simulink model "Tetris"  (R2023a)
settings: Solver=VariableStepAuto  StartTime=0.0  StopTime=inf  RelTol=1e-3  EnableMultiTasking=on
libraries: Miscellaneous x183, Byte_Multiplexers_Lib x77, Tetris_Lib x34, simulink_extras x11, Counters_Lib x7, Arithmetic_Operations_Lib x5, Word_Multiplexers_Lib x5, Decoders_Lib x4, Memory_Blocks_Lib x3, Bit_Multiplexers_Lib x2, dspobslib x1
(part 1 of 3)
settings Model: SnapshotBufferSize=2000  SnapshotInterval=1  PacingRate=79  Creator=Jozko Mrkvicka  LastModifiedBy=Jozko Mrkvicka
settings SolverCC: AlgebraicLoopSolver=TrustRegion
settings DataIOCC: ReturnWorkspaceOutputs=off
settings OptimizationCC: LifeSpan=inf
settings DebuggingCC: UnconnectedInputMsg=warning  UnconnectedOutputMsg=warning  UnconnectedLineMsg=warning  SFUnexpectedBacktrackingDiag=warning  SFNoUnconditionalDefaultTransitionDiag=warning  ArithmeticOperatorsInVariantConditions=warning
settings ModelReferenceCC: EnableRefExpFcnMdlSchedulingChecks=on
settings SFSimCC: SimUseLocalCustomCode=off  CustomCodeUndefinedFunction=UseInterfaceOnly
settings RTWCC: RTWUseLocalCustomCode=off
settings CodeAppCC: StateflowObjectComments=on
settings GRTTargetCC: TargetLangStandard=C89/C90 (ANSI)
settings ConfigComp: CovMetricSettings=dw  CovSaveCumulativeToWorkspaceVar=on  CovSaveSingleToWorkspaceVar=on  CovExternalEMLEnable=off

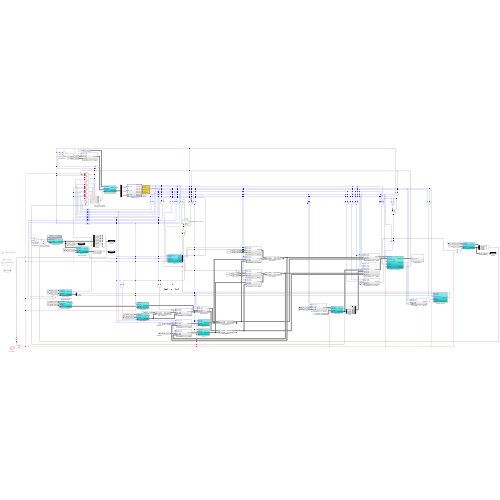
[thumbnail: Simulink's stored preview of the top-level diagram]
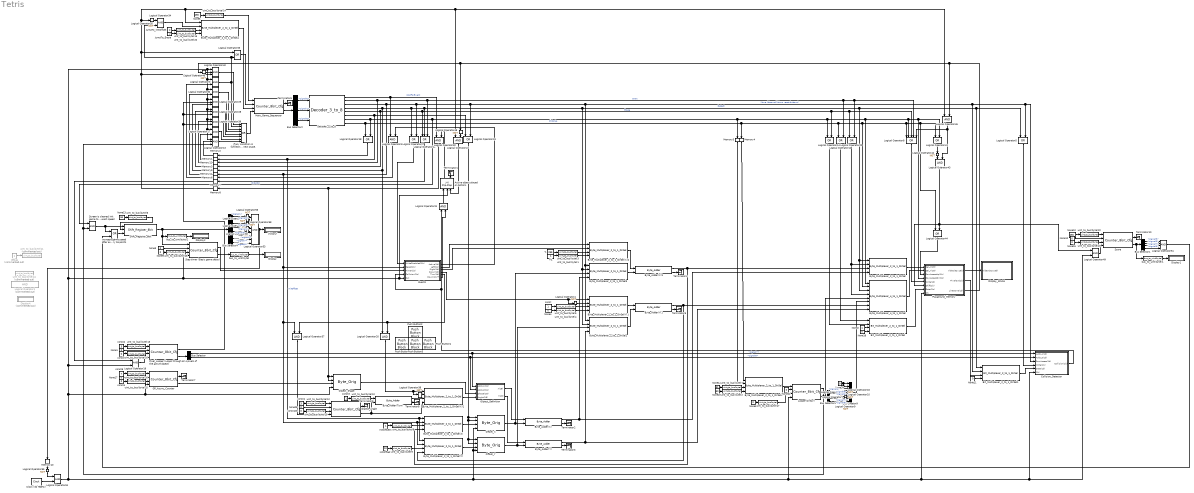
== system Tetris ==
  +1 : Constant  OutDataTypeStr=uint8
  -1 : Constant  Value=255  OutDataTypeStr=uint8
  "Active object placed on bottom " : simulink_extras/Flip Flops/J-K Flip-Flop  initial_condition=0
  Bit_Multiplexer_2_to_1_DirSel : Bit_Multiplexers_Lib/Bit_Multiplexers_Lib/Bit_Multiplexer_2_to_1_DirSel  SystemSampleTime=-1  VariantActivationTime=update diagram  Latency=0  AutoFrameSizeCalculation=off
  Bit_Multiplexer_2_to_1_DirSel1 : Bit_Multiplexers_Lib/Bit_Multiplexers_Lib/Bit_Multiplexer_2_to_1_DirSel  SystemSampleTime=-1  VariantActivationTime=update diagram  Latency=0  AutoFrameSizeCalculation=off
  Bus Creator9 : BusCreator  Inputs=8
  Bus Selector : BusSelector  OutputSignals=signal7,signal8
  Bus Selector1 : BusSelector  OutputSignals=signal5,signal6,signal7,signal8
  Bus Selector2 : BusSelector  OutputSignals=signal6,signal7,signal8
  Bus Selector3 : BusSelector  OutputSignals=signal4,signal5,signal6,signal7,signal8
  Bus Selector4 : BusSelector  OutputSignals=signal1,signal2,signal3,signal4,signal5,signal6,signal7,signal8
  Byte_Adder(Turn) : Arithmetic_Operations_Lib/Arithmetic_Operations_Lib/Byte_Adder  SystemSampleTime=-1  VariantActivationTime=update diagram  Latency=0  AutoFrameSizeCalculation=off
  Byte_Adder(X) : Arithmetic_Operations_Lib/Arithmetic_Operations_Lib/Byte_Adder  SystemSampleTime=-1  VariantActivationTime=update diagram  Latency=0  AutoFrameSizeCalculation=off
  Byte_Adder(X)1 : Arithmetic_Operations_Lib/Arithmetic_Operations_Lib/Byte_Adder  SystemSampleTime=-1  VariantActivationTime=update diagram  Latency=0  AutoFrameSizeCalculation=off
  Byte_Adder(Y) : Arithmetic_Operations_Lib/Arithmetic_Operations_Lib/Byte_Adder  SystemSampleTime=-1  VariantActivationTime=update diagram  Latency=0  AutoFrameSizeCalculation=off
  Byte_Adder(Y)1 : Arithmetic_Operations_Lib/Arithmetic_Operations_Lib/Byte_Adder  SystemSampleTime=-1  VariantActivationTime=update diagram  Latency=0  AutoFrameSizeCalculation=off
  Byte_Multiplexer_2_to_1_DirSel{,1..4} (5 alike) : Byte_Multiplexers_Lib/Byte_Multiplexers_Lib/Byte_Multiplexer_2_to_1_DirSel  SystemSampleTime=-1  VariantActivationTime=update diagram  Latency=0  AutoFrameSizeCalculation=off
  Byte_Multiplexer_2_to_1_DirSel(X) : Byte_Multiplexers_Lib/Byte_Multiplexers_Lib/Byte_Multiplexer_2_to_1_DirSel  SystemSampleTime=-1  VariantActivationTime=update diagram  Latency=0  AutoFrameSizeCalculation=off
  Byte_Multiplexer_2_to_1_DirSel(X)1 : Byte_Multiplexers_Lib/Byte_Multiplexers_Lib/Byte_Multiplexer_2_to_1_DirSel  SystemSampleTime=-1  VariantActivationTime=update diagram  Latency=0  AutoFrameSizeCalculation=off
  Byte_Multiplexer_2_to_1_DirSel(X)2 : Byte_Multiplexers_Lib/Byte_Multiplexers_Lib/Byte_Multiplexer_2_to_1_DirSel  SystemSampleTime=-1  VariantActivationTime=update diagram  Latency=0  AutoFrameSizeCalculation=off
  Byte_Multiplexer_2_to_1_DirSel(Y) : Byte_Multiplexers_Lib/Byte_Multiplexers_Lib/Byte_Multiplexer_2_to_1_DirSel  SystemSampleTime=-1  VariantActivationTime=update diagram  Latency=0  AutoFrameSizeCalculation=off
  Byte_Multiplexer_2_to_1_DirSel(Y)1 : Byte_Multiplexers_Lib/Byte_Multiplexers_Lib/Byte_Multiplexer_2_to_1_DirSel  SystemSampleTime=-1  VariantActivationTime=update diagram  Latency=0  AutoFrameSizeCalculation=off
  Byte_Multiplexer_4_to_1_DirSel : Byte_Multiplexers_Lib/Byte_Multiplexers_Lib/Byte_Multiplexer_4_to_1_DirSel  SystemSampleTime=-1  VariantActivationTime=update diagram  Latency=0  AutoFrameSizeCalculation=off
  Clock (32 768Hz) : simulink_extras/Flip Flops/Clock  period=1
  Collision_Detector : Subsystem
  Decoder_3_to_8 : Decoders_Lib/Decoders_Lib/Decoder_3_to_8  SystemSampleTime=-1  VariantActivationTime=update diagram  Latency=0  AutoFrameSizeCalculation=off
  Display : Display
  Display1 : Display
  Display2 : Display
  Display4 : Display  Commented=on
  Display_32x16 : Subsystem
  Events : Subsystem
  GP_Async_Counter : Counters_Lib/Counter_8bit_Cfg  SystemSampleTime=-1  VariantActivationTime=update diagram  Latency=0  AutoFrameSizeCalculation=off
  If any condition is fulfilled then we go to next state. : Logic  Operator=OR  Inputs=8  IconShape=distinctive  AllPortsSameDT=off  OutDataTypeStr=boolean
  Increase game speed after every 16 points : Logic  Operator=OR  IconShape=distinctive  OutDataTypeStr=boolean
  InitOffsetX : Constant  OutDataTypeStr=uint8
  InitOffsetY : Constant  Value=10  OutDataTypeStr=uint8
  "JumpTo_Erase     " : Constant  Value=3  OutDataTypeStr=uint8
  JumpTo_InitOffset : Constant  Value=2  OutDataTypeStr=uint8
  Logical Operator1 : Logic  Commented=on  Inputs=12  IconShape=distinctive  AllPortsSameDT=off  OutDataTypeStr=boolean
  Logical Operator{4,7,9..11,16,35,42,46,48,55..60} (16 alike) : Logic  Operator=NOT  Inputs=4  IconShape=distinctive  AllPortsSameDT=off  OutDataTypeStr=boolean
  Logical Operator{5,12,14,18,22..23,27,33,41,44} (10 alike) : Logic  Operator=OR  IconShape=distinctive  OutDataTypeStr=boolean
  Logical Operator{13,28..29,39..40} (5 alike) : Logic  Inputs=3  IconShape=distinctive  AllPortsSameDT=off  OutDataTypeStr=boolean
  Logical Operator{3,6,17,20,30..32,34,37,43,45,47,49,61} (14 alike) : Logic  IconShape=distinctive  AllPortsSameDT=off  OutDataTypeStr=boolean
  Logical Operator19 : Logic  IconShape=distinctive  AllPortsSameDT=off
  Logical Operator21 : Logic  Operator=OR  Inputs=3  IconShape=distinctive  AllPortsSameDT=off  OutDataTypeStr=boolean
  Logical Operator38 : Logic  Operator=NOT  IconShape=distinctive  AllPortsSameDT=off  OutDataTypeStr=boolean
  Logical Operator51 : Logic  Inputs=4  IconShape=distinctive  AllPortsSameDT=off  OutDataTypeStr=boolean
  Logical Operator53 : Logic  Inputs=8  IconShape=distinctive  AllPortsSameDT=off  OutDataTypeStr=boolean
  Logical Operator8 : Logic  Operator=OR  Inputs=5  IconShape=distinctive  OutDataTypeStr=boolean
  Looper(ClrScr) : Counters_Lib/Counter_8bit_Cfg  SystemSampleTime=-1  VariantActivationTime=update diagram  Latency=0  AutoFrameSizeCalculation=off
  Main_Game_Sequencer : Counters_Lib/Counter_8bit_Cfg  SystemSampleTime=-1  VariantActivationTime=update diagram  Latency=0  AutoFrameSizeCalculation=off
  Memory{1..12} (12 alike) : Memory
  None{1,3,11..12,17..18,22,24,28} (9 alike) : Constant  Value=0  OutDataTypeStr=boolean
  None10 : Constant  Value=255  OutDataTypeStr=uint8
  None13 : Constant  Value=64  OutDataTypeStr=uint8
  None14 : Constant  Value=31  OutDataTypeStr=uint8
  None{4,8..9,15} (4 alike) : Constant  Value=0  OutDataTypeStr=uint8
  None2 : Constant  OutDataTypeStr=boolean
  None23 : Constant  Value=30  OutDataTypeStr=uint8
  None5 : Constant  Value=255  OutDataTypeStr=uint8
  Object_Angle : Counters_Lib/Counter_8bit_Cfg  SystemSampleTime=-1  VariantActivationTime=update diagram  Latency=0  AutoFrameSizeCalculation=off
  Object_Definition : Subsystem
  Object_Shape : Memory_Blocks_Lib/Memory_Blocks_Lib/Byte_Orig  SystemSampleTime=-1  VariantActivationTime=update diagram  Latency=0  AutoFrameSizeCalculation=off
  Offset_X : Memory_Blocks_Lib/Memory_Blocks_Lib/Byte_Orig  SystemSampleTime=-1  VariantActivationTime=update diagram  Latency=0  AutoFrameSizeCalculation=off
  Offset_Y : Memory_Blocks_Lib/Memory_Blocks_Lib/Byte_Orig  SystemSampleTime=-1  VariantActivationTime=update diagram  Latency=0  AutoFrameSizeCalculation=off
  Pixel_Looper (Loops through all 4 pixels of the active object) : Counters_Lib/Counter_8bit_Cfg  SystemSampleTime=-1  VariantActivationTime=update diagram  Latency=0  AutoFrameSizeCalculation=off
  Playground_Memory : Subsystem
  Push Button : PushButtonBlock  ButtonText=Left  OffValue=0.000000
  Push Button1 : PushButtonBlock  ButtonText=Right  OffValue=0.000000
  Push Button2 : PushButtonBlock  ButtonText=Turn  OffValue=0.000000
  Push Button3 : PushButtonBlock  ButtonText=Down  OffValue=0.000000
  Score : Counters_Lib/Counter_8bit_Cfg  SystemSampleTime=-1  VariantActivationTime=update diagram  Latency=0  AutoFrameSizeCalculation=off
  Screen is cleared; Init game to slowest speed : Logic  IconShape=distinctive  AllPortsSameDT=off  OutDataTypeStr=boolean
  Shift_Register_8bit : Tetris_Lib/Shift_Register_8bit  SystemSampleTime=-1  VariantActivationTime=update diagram  Latency=0  AutoFrameSizeCalculation=off
  Step timer (Basic game delay) : Counters_Lib/Counter_8bit_Cfg  SystemSampleTime=-1  VariantActivationTime=update diagram  Latency=0  AutoFrameSizeCalculation=off
  Terminator{1..10} (10 alike) : Terminator
  Victory! : Display
  bus_to_uint(byte) : Miscellaneous/bus_to_uint(byte)  SystemSampleTime=-1  VariantActivationTime=update diagram  Latency=0  AutoFrameSizeCalculation=off
  bus_to_uint(byte)1 : Miscellaneous/bus_to_uint(byte)  SystemSampleTime=-1  VariantActivationTime=update diagram  Latency=0  AutoFrameSizeCalculation=off
  bus_to_uint(byte)2 : Miscellaneous/bus_to_uint(byte)  SystemSampleTime=-1  VariantActivationTime=update diagram  Latency=0  AutoFrameSizeCalculation=off
  const : Constant  OutDataTypeStr=uint8
  const1 : Constant  Value=3  OutDataTypeStr=uint8
  const100 : Constant  Value=0  OutDataTypeStr=uint8
  const2 : Constant  Value=3  OutDataTypeStr=uint8
  const3 : Constant  OutDataTypeStr=uint8
  const4 : Constant  Value=0  OutDataTypeStr=uint8
  const5 : Constant  Value=0  OutDataTypeStr=uint8
  const6 : Constant  Value=7  OutDataTypeStr=uint8
  debug : Constant  Commented=on  OutDataTypeStr=uint8
  uint_to_bus(byte){1..10,12..20,22..23,25..26} (23 alike) : Miscellaneous/uint_to_bus(byte)  SystemSampleTime=-1  VariantActivationTime=update diagram  Latency=0  AutoFrameSizeCalculation=off
  uint_to_bus(byte)11 : Miscellaneous/uint_to_bus(byte)  Commented=on  SystemSampleTime=-1  VariantActivationTime=update diagram  Latency=0  AutoFrameSizeCalculation=off
  uint_to_bus(byte)24 : Miscellaneous/uint_to_bus(byte)  Commented=on  SystemSampleTime=-1  VariantActivationTime=update diagram  Latency=0  AutoFrameSizeCalculation=off
  wires:
  None1/1 -> Pixel_Looper (Loops through all 4 pixels of the active object)/2
  Playground_Memory/2(PixelOut(1b)) -> Bit_Multiplexer_2_to_1_DirSel1/3
  Playground_Memory/1(Video(32x16b)) -> Display_32x16/1(Video(32x16b))
  Offset_Y/1 -> Byte_Multiplexer_2_to_1_DirSel2/3, Byte_Adder(Y)/2
  Offset_X/1 -> Byte_Multiplexer_2_to_1_DirSel3/3, Byte_Adder(X)/2
  Bit_Multiplexer_2_to_1_DirSel/1 -> Playground_Memory/7(Data(1b))
  Pixel_Looper (Loops through all 4 pixels of the active object)/2 -> Bus Selector/1
  uint_to_bus(byte)13/1 -> Pixel_Looper (Loops through all 4 pixels of the active object)/1
  Byte_Adder(X)/2 -> Terminator2/1
  Byte_Adder(Y)/2 -> Terminator3/1
  uint_to_bus(byte)4/1 -> Byte_Multiplexer_2_to_1_DirSel(Y)1/4
  uint_to_bus(byte)5/1 -> Byte_Multiplexer_2_to_1_DirSel(Y)1/3
  Bus Selector/1 -> Collision_Detector/1(Addr_1(1b)), Object_Definition/1(Addr_1(1b))  "<signal7>"
  Bus Selector/2 -> Collision_Detector/2(Addr_0(1b)), Object_Definition/2(Addr_0(1b))  "<signal8>"
  Decoder_3_to_8/4 -> Logical Operator5/1, Bit_Multiplexer_2_to_1_DirSel1/1, Byte_Multiplexer_4_to_1_DirSel/3, Byte_Multiplexer_2_to_1_DirSel/1, Byte_Multiplexer_2_to_1_DirSel3/2, Byte_Multiplexer_2_to_1_DirSel2/2, Logical Operator21/2, Logical Operator27/1, Memory9/1, Logical Operator20/1  "Detect"
  Decoder_3_to_8/3 -> Collision_Detector/3(RowAccess(1b)), Logical Operator5/2, Bit_Multiplexer_2_to_1_DirSel1/2, Byte_Multiplexer_2_to_1_DirSel2/1, Byte_Multiplexer_2_to_1_DirSel3/1, Logical Operator23/2, Logical Operator27/2, Logical Operator37/1, Byte_Multiplexer_2_to_1_DirSel(X)/2, Byte_Multiplexer_2_to_1_DirSel(Y)/2, Events/2(Reset(1b)), Memory11/1  "Move (clear collisions, reset buttons)"
  None2/1 -> Bit_Multiplexer_2_to_1_DirSel/3
  None18/1 -> Bit_Multiplexer_2_to_1_DirSel/4
  Logical Operator8/1 -> Playground_Memory/5(Write(1b))
  Decoder_3_to_8/5 -> Logical Operator8/3, Logical Operator22/1, Logical Operator14/2, Logical Operator21/1, Memory3/1  "Erase"
  Byte_Multiplexer_2_to_1_DirSel(X)2/1 -> Byte_Adder(X)1/1
  Byte_Multiplexer_2_to_1_DirSel(Y)1/1 -> Byte_Adder(Y)1/1
  Byte_Multiplexer_2_to_1_DirSel/1 -> Playground_Memory/1(Sel_X(1B))
  Byte_Multiplexer_4_to_1_DirSel/1 -> Playground_Memory/2(Sel_Y(1B))
  Byte_Adder(X)/1 -> Byte_Multiplexer_2_to_1_DirSel3/4, Byte_Multiplexer_2_to_1_DirSel/4
  Byte_Adder(Y)/1 -> Byte_Multiplexer_2_to_1_DirSel2/4, Byte_Multiplexer_4_to_1_DirSel/8
  Object_Definition/1(X(1B)) -> Byte_Adder(X)/1
  Object_Definition/2(Y(1B)) -> Byte_Adder(Y)/1
  Byte_Multiplexer_2_to_1_DirSel(Y)/1 -> Offset_Y/3
  Byte_Multiplexer_2_to_1_DirSel(X)/1 -> Offset_X/3
  None11/1 -> Bit_Multiplexer_2_to_1_DirSel1/4
  Logical Operator5/1 -> Collision_Detector/4(Write(1b))
  Bus Selector2/2 -> Decoder_3_to_8/2  "<signal7>"
  Main_Game_Sequencer/2 -> Bus Selector2/1
  Bus Selector2/3 -> Decoder_3_to_8/3  "<signal8>"
  Decoder_3_to_8/6 -> Logical Operator23/1, Memory1/1, Byte_Multiplexer_2_to_1_DirSel(X)/1, Byte_Multiplexer_2_to_1_DirSel(Y)/1  "InitOffset"
  Decoder_3_to_8/8 -> Memory4/1, Byte_Multiplexer_4_to_1_DirSel/2, Logical Operator44/1, Logical Operator41/1, Logical Operator8/1, Logical Operator12/1, Logical Operator18/1  "ClrScrUp"
  If any condition is fulfilled then we go to next state./1 -> Main_Game_Sequencer/4
  None23/1 -> uint_to_bus(byte)2/1
  None22/1 -> Looper(ClrScr)/2
  None24/1 -> Bus Creator9/3, Bus Creator9/2, Bus Creator9/1
  Bus Creator9/1 -> Byte_Multiplexer_4_to_1_DirSel/6
  Decoder_3_to_8/7 -> Screen is cleared; Init game to slowest speed/1, Byte_Multiplexer_4_to_1_DirSel/1, Logical Operator41/2, Playground_Memory/4(RowAccessDn(1b)), Logical Operator8/2, Logical Operator14/1, Memory5/1, Logical Operator18/2  "ClrScrDn"
  Logical Operator9/1 -> Bus Creator9/8
  Logical Operator7/1 -> Bus Creator9/7
  Logical Operator10/1 -> Bus Creator9/6
  Logical Operator11/1 -> Bus Creator9/5
  Logical Operator13/1 -> If any condition is fulfilled then we go to next state./8
  Looper(ClrScr)/1 -> Logical Operator13/3, Screen is cleared; Init game to slowest speed/2
  Collision_Detector/1(Collision(1b)) -> Events/4(Collision(1b)), Logical Operator31/1
  Logical Operator12/1 -> Bit_Multiplexer_2_to_1_DirSel/1
  Looper(ClrScr)/2 -> Byte_Multiplexer_4_to_1_DirSel/5, Bus Selector3/1
  Logical Operator14/1 -> Bit_Multiplexer_2_to_1_DirSel/2
  Logical Operator16/1 -> Bus Creator9/4
  Bus Selector3/1 -> Logical Operator16/1  "<signal4>"
  Bus Selector3/2 -> Logical Operator11/1  "<signal5>"
  Bus Selector3/3 -> Logical Operator10/1  "<signal6>"
  Bus Selector3/4 -> Logical Operator7/1  "<signal7>"
  Bus Selector3/5 -> Logical Operator9/1  "<signal8>"
  Logical Operator17/1 -> If any condition is fulfilled then we go to next state./7
  Logical Operator18/1 -> Memory2/1
  Logical Operator19/1 -> Pixel_Looper (Loops through all 4 pixels of the active object)/4
  Logical Operator22/1 -> Byte_Multiplexer_4_to_1_DirSel/4, Byte_Multiplexer_2_to_1_DirSel/2
  Logical Operator4/1 -> Byte_Multiplexer_2_to_1_DirSel(Y)1/2
  +1/1 -> uint_to_bus(byte)1/1
  uint_to_bus(byte)1/1 -> Byte_Multiplexer_2_to_1_DirSel(X)2/4
  -1/1 -> uint_to_bus(byte)3/1
  uint_to_bus(byte)3/1 -> Byte_Multiplexer_2_to_1_DirSel(X)2/3
  None4/1 -> uint_to_bus(byte)4/1
  const/1 -> uint_to_bus(byte)5/1
  uint_to_bus(byte)6/1 -> Shift_Register_8bit/2
  None13/1 -> uint_to_bus(byte)6/1
  None3/1 -> Step timer (Basic game delay)/2
  Byte_Multiplexer_2_to_1_DirSel1/1 -> Looper(ClrScr)/1
  uint_to_bus(byte)2/1 -> Byte_Multiplexer_2_to_1_DirSel1/4
  None14/1 -> uint_to_bus(byte)7/1
  uint_to_bus(byte)7/1 -> Byte_Multiplexer_2_to_1_DirSel1/3
  Memory4/1 -> Byte_Multiplexer_2_to_1_DirSel1/1
  Memory5/1 -> Byte_Multiplexer_2_to_1_DirSel1/2
  None28/1 -> Object_Angle/2
  InitOffsetX/1 -> uint_to_bus(byte)8/1
  InitOffsetY/1 -> uint_to_bus(byte)9/1
  uint_to_bus(byte)8/1 -> Byte_Multiplexer_2_to_1_DirSel(X)/3
  uint_to_bus(byte)9/1 -> Byte_Multiplexer_2_to_1_DirSel(Y)/3
  Pixel_Looper (Loops through all 4 pixels of the active object)/1 -> Logical Operator39/3, Logical Operator28/3, Logical Operator29/2
  Memory7/1 -> Logical Operator19/1
  Logical Operator21/1 -> Memory7/1
  Events/2(Left(1b)) -> Byte_Multiplexer_2_to_1_DirSel(X)2/1
  Events/3(Right(1b)) -> Byte_Multiplexer_2_to_1_DirSel(X)2/2
  Bit_Multiplexer_2_to_1_DirSel1/1 -> Collision_Detector/5(Data(1b))
  Logical Operator23/1 -> Offset_Y/2, Offset_Y/1, Offset_X/2, Offset_X/1
  Logical Operator27/1 -> Events/1(WriteDisabled(1b))
  Byte_Adder(Y)1/1 -> Byte_Multiplexer_4_to_1_DirSel/7, Byte_Multiplexer_2_to_1_DirSel(Y)/4
  Byte_Adder(X)1/1 -> Byte_Multiplexer_2_to_1_DirSel/3, Byte_Multiplexer_2_to_1_DirSel(X)/4
  Byte_Adder(X)1/2 -> Terminator4/1
  Byte_Adder(Y)1/2 -> Terminator5/1
  Byte_Multiplexer_2_to_1_DirSel3/1 -> Byte_Adder(X)1/2
  Byte_Multiplexer_2_to_1_DirSel2/1 -> Byte_Adder(Y)1/2
  Decoder_3_to_8/2 -> Memory12/1, Logical Operator12/2, Logical Operator22/2, Logical Operator8/4, Logical Operator21/3  "Draw"
  Bus Selector2/1 -> Decoder_3_to_8/1  "<signal6>"
  Events/4(Down(1b)) -> Byte_Multiplexer_2_to_1_DirSel(Y)1/1, Logical Operator4/1
  Events/5(Turn(1b)) -> Logical Operator37/2, Logical Operator20/2
  const3/1 -> uint_to_bus(byte)10/1
  uint_to_bus(byte)10/1 -> Byte_Adder(Turn)/1
  Object_Angle/2 -> Byte_Adder(Turn)/2, Byte_Multiplexer_2_to_1_DirSel(X)1/4
  Byte_Adder(Turn)/2 -> Terminator8/1
  Byte_Adder(Turn)/1 -> Byte_Multiplexer_2_to_1_DirSel(X)1/3
  Byte_Multiplexer_2_to_1_DirSel(X)1/1 -> Object_Definition/4(Angle(1B))
  Logical Operator37/1 -> Object_Angle/4
  Logical Operator20/1 -> Logical Operator38/1, Byte_Multiplexer_2_to_1_DirSel(X)1/1
  Logical Operator38/1 -> Byte_Multiplexer_2_to_1_DirSel(X)1/2
  Logical Operator61/1 -> Logical Operator19/2, Logical Operator40/1, Logical Operator13/1, Logical Operator17/1, Logical Operator39/1, Logical Operator28/1, Logical Operator29/1, Logical Operator30/1, Logical Operator3/1, Step timer (Basic game delay)/4, "Active object placed on bottom "/2, Events/5(CLK), Object_Shape/4, GP_Async_Counter/4, Looper(ClrScr)/4, Collision_Detector/6(CLK), Logical Operator49/2, Playground_Memory/8(Clk), Offset_X/4, Offset_Y/4
  const1/1 -> uint_to_bus(byte)12/1
  uint_to_bus(byte)12/1 -> Object_Angle/1
  Object_Angle/1 -> Terminator9/1
  const2/1 -> uint_to_bus(byte)13/1
  None5/1 -> uint_to_bus(byte)14/1
  uint_to_bus(byte)14/1 -> Main_Game_Sequencer/1
  Byte_Multiplexer_2_to_1_DirSel4/1 -> Main_Game_Sequencer/3
  "JumpTo_Erase     "/1 -> uint_to_bus(byte)20/1
  const5/1 -> uint_to_bus(byte)16/1
  uint_to_bus(byte)16/1 -> Pixel_Looper (Loops through all 4 pixels of the active object)/3
  None8/1 -> uint_to_bus(byte)17/1
  uint_to_bus(byte)17/1 -> Looper(ClrScr)/3
  uint_to_bus(byte)18/1 -> Step timer (Basic game delay)/3
  None9/1 -> uint_to_bus(byte)18/1
  const100/1 -> uint_to_bus(byte)19/1
  uint_to_bus(byte)19/1 -> Object_Angle/3
  Logical Operator28/1 -> If any condition is fulfilled then we go to next state./5
  Logical Operator29/1 -> If any condition is fulfilled then we go to next state./4
  Logical Operator30/1 -> If any condition is fulfilled then we go to next state./3
  Memory2/1 -> Logical Operator13/2
  Memory12/1 -> Logical Operator39/2
  Memory3/1 -> Logical Operator28/2
  Memory9/1 -> Logical Operator29/3
  Memory1/1 -> Logical Operator17/2
  Decoder_3_to_8/1 -> Logical Operator32/1, Logical Operator6/1  "WaitForEvent"
  Main_Game_Sequencer/1 -> Terminator6/1
  Memory11/1 -> Logical Operator30/2
  Step timer (Basic game delay)/2 -> bus_to_uint(byte)/1
  Logical Operator6/1 -> Memory6/1
  Logical Operator3/1 -> Logical Operator33/2, Logical Operator34/2, If any condition is fulfilled then we go to next state./2
  Logical Operator39/1 -> If any condition is fulfilled then we go to next state./6
  Step timer (Basic game delay)/1 -> Events/3(Timer(1b))
  bus_to_uint(byte)/1 -> Display/1
  Events/1(Active(1b)) -> Logical Operator6/2
  Memory6/1 -> Logical Operator3/2
  Logical Operator31/1 -> "Active object placed on bottom "/1
  "Active object placed on bottom "/1 -> Logical Operator32/2
  JumpTo_InitOffset/1 -> uint_to_bus(byte)15/1
  uint_to_bus(byte)15/1 -> Byte_Multiplexer_2_to_1_DirSel4/3
  uint_to_bus(byte)20/1 -> Byte_Multiplexer_2_to_1_DirSel4/4
  Logical Operator33/1 -> Main_Game_Sequencer/2
  Logical Operator34/1 -> Byte_Multiplexer_2_to_1_DirSel4/2
  Logical Operator35/1 -> Logical Operator34/1
  Logical Operator40/1 -> If any condition is fulfilled then we go to next state./1
  Playground_Memory/3(LineDone(1b)) -> Logical Operator46/1, Logical Operator48/1, Logical Operator45/2
  Logical Operator41/1 -> Logical Operator42/1
  Logical Operator42/1 -> Logical Operator43/1
  Logical Operator44/1 -> Playground_Memory/3(RowAccessUp(1b))
  Logical Operator45/1 -> Logical Operator8/5, Logical Operator43/2
  Logical Operator46/1 -> Logical Operator40/2
  Logical Operator47/1 -> "Active object placed on bottom "/3
  Logical Operator48/1 -> Logical Operator47/2
  None10/1 -> uint_to_bus(byte)22/1
  uint_to_bus(byte)22/1 -> Score/1
  None12/1 -> Score/2
  bus_to_uint(byte)1/1 -> Display1/1
  Score/2 -> bus_to_uint(byte)1/1, Bus Selector1/1
  Logical Operator43/1 -> Playground_Memory/6(Shift(1b)), Logical Operator49/1, Logical Operator44/2
  uint_to_bus(byte)23/1 -> Score/3
  None15/1 -> uint_to_bus(byte)23/1
  Logical Operator49/1 -> Score/4
  Shift_Register_8bit/1 -> Step timer (Basic game delay)/1, bus_to_uint(byte)2/1, Bus Selector4/1
  Screen is cleared; Init game to slowest speed/1 -> Shift_Register_8bit/1, Increase game speed after every 16 points/1
  Bus Selector1/1 -> Logical Operator51/1  "<signal5>"
  Bus Selector1/3 -> Logical Operator51/3  "<signal7>"
  Bus Selector1/2 -> Logical Operator51/2  "<signal6>"
  Bus Selector1/4 -> Logical Operator51/4  "<signal8>"
  Logical Operator51/1 -> Increase game speed after every 16 points/2
  Increase game speed after every 16 points/1 -> Shift_Register_8bit/3
  bus_to_uint(byte)2/1 -> Display2/1
  Bus Selector4/1 -> Logical Operator56/1  "<signal1>"
  Bus Selector4/2 -> Logical Operator57/1  "<signal2>"
  Bus Selector4/3 -> Logical Operator58/1  "<signal3>"
  Bus Selector4/4 -> Logical Operator59/1  "<signal4>"
  Logical Operator56/1 -> Logical Operator53/1
  Logical Operator57/1 -> Logical Operator53/2
  Logical Operator58/1 -> Logical Operator53/3
  Logical Operator59/1 -> Logical Operator53/4
  Bus Selector4/5 -> Logical Operator60/1  "<signal5>"
  Bus Selector4/6 -> Logical Operator53/6  "<signal6>"
  Bus Selector4/7 -> Logical Operator53/7  "<signal7>"
  Bus Selector4/8 -> Logical Operator53/8  "<signal8>"
  Logical Operator60/1 -> Logical Operator53/5
  Logical Operator53/1 -> Victory!/1, Memory10/1
  Clock (32 768Hz)/1 -> Logical Operator61/2
  Logical Operator55/1 -> Logical Operator61/1
  Memory10/1 -> Logical Operator55/1
  Memory8/1 -> Logical Operator45/1, Logical Operator47/1, Byte_Multiplexer_2_to_1_DirSel4/1, Logical Operator35/1, Logical Operator33/1, Logical Operator40/3
  "Active object placed on bottom "/2 -> Terminator1/1
  Object_Shape/1 -> Object_Definition/3(Shape(1B))
  debug/1 -> uint_to_bus(byte)11/1
  const4/1 -> uint_to_bus(byte)25/1
  None17/1 -> GP_Async_Counter/2
  uint_to_bus(byte)25/1 -> GP_Async_Counter/3
  uint_to_bus(byte)26/1 -> GP_Async_Counter/1
  const6/1 -> uint_to_bus(byte)26/1
  GP_Async_Counter/2 -> Object_Shape/3
  GP_Async_Counter/1 -> Terminator7/1
  Score/1 -> Terminator10/1
  Logical Operator32/1 -> Memory8/1, Object_Shape/1, Object_Shape/2
  Events/6(Down(1b)+) -> Logical Operator31/2

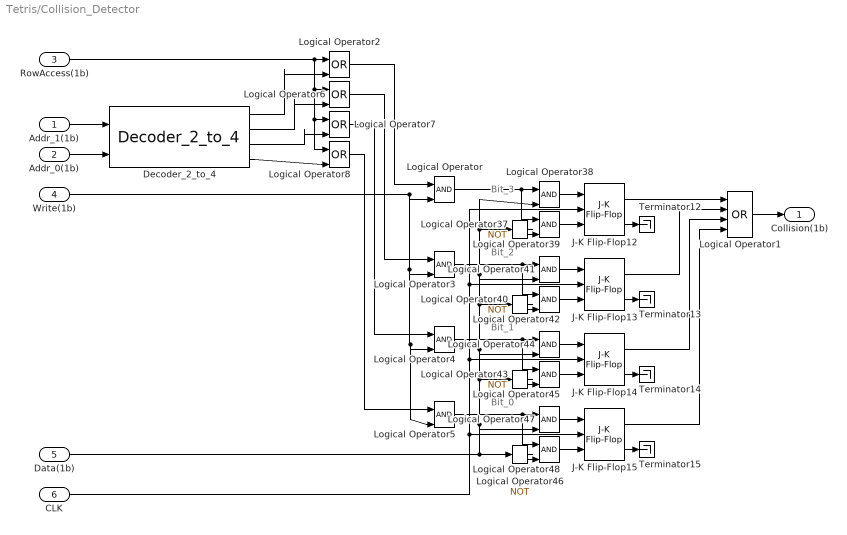
== system Tetris/Collision_Detector ==
  note: Bit_0
  note: Bit_1
  note: Bit_2
  note: Bit_3
  Addr_1(1b) : Inport
  Addr_0(1b) : Inport  Port=2
  RowAccess(1b) : Inport  Port=3
  Write(1b) : Inport  Port=4
  Data(1b) : Inport  Port=5
  CLK : Inport  Port=6
  Decoder_2_to_4 : Decoders_Lib/Decoders_Lib/Decoder_2_to_4  SystemSampleTime=-1  VariantActivationTime=update diagram  Latency=0  AutoFrameSizeCalculation=off
  J-K Flip-Flop{12..15} (4 alike) : simulink_extras/Flip Flops/J-K Flip-Flop  initial_condition=0
  Logical Operator{,3..5,38..39,41..42,44..45,47..48} (12 alike) : Logic  IconShape=distinctive  AllPortsSameDT=off  OutDataTypeStr=boolean
  Logical Operator1 : Logic  Operator=OR  Inputs=4  IconShape=distinctive  AllPortsSameDT=off  OutDataTypeStr=boolean
  Logical Operator{2,6..8} (4 alike) : Logic  Operator=OR  IconShape=distinctive  AllPortsSameDT=off  OutDataTypeStr=boolean
  Logical Operator{37,40,43,46} (4 alike) : Logic  Operator=NOT  IconShape=distinctive  AllPortsSameDT=off  OutDataTypeStr=boolean
  Terminator{12..15} (4 alike) : Terminator
  Collision(1b) : Outport
  wires:
  Logical Operator38/1 -> J-K Flip-Flop12/1
  J-K Flip-Flop12/2 -> Terminator12/1
  CLK/1 -> J-K Flip-Flop15/2, J-K Flip-Flop14/2, J-K Flip-Flop12/2, J-K Flip-Flop13/2
  Logical Operator37/1 -> Logical Operator39/2
  Logical Operator43/1 -> Logical Operator45/2
  J-K Flip-Flop14/1 -> Logical Operator1/3
  Logical Operator39/1 -> J-K Flip-Flop12/3
  J-K Flip-Flop12/1 -> Logical Operator1/1
  J-K Flip-Flop13/1 -> Logical Operator1/2
  Logical Operator42/1 -> J-K Flip-Flop13/3
  Logical Operator40/1 -> Logical Operator42/2
  Logical Operator47/1 -> J-K Flip-Flop15/1
  Logical Operator45/1 -> J-K Flip-Flop14/3
  Logical Operator44/1 -> J-K Flip-Flop14/1
  Data(1b)/1 -> Logical Operator38/2, Logical Operator37/1, Logical Operator41/2, Logical Operator40/1, Logical Operator44/2, Logical Operator43/1, Logical Operator47/2, Logical Operator46/1
  Logical Operator48/1 -> J-K Flip-Flop15/3
  J-K Flip-Flop15/2 -> Terminator15/1
  J-K Flip-Flop15/1 -> Logical Operator1/4
  J-K Flip-Flop14/2 -> Terminator14/1
  Write(1b)/1 -> Logical Operator/2, Logical Operator3/2, Logical Operator4/2, Logical Operator5/2
  J-K Flip-Flop13/2 -> Terminator13/1
  Logical Operator41/1 -> J-K Flip-Flop13/1
  Logical Operator46/1 -> Logical Operator48/2
  Logical Operator1/1 -> Collision(1b)/1
  Addr_0(1b)/1 -> Decoder_2_to_4/2
  Addr_1(1b)/1 -> Decoder_2_to_4/1
  Logical Operator5/1 -> Logical Operator47/1, Logical Operator48/1
  Logical Operator4/1 -> Logical Operator44/1, Logical Operator45/1
  Logical Operator3/1 -> Logical Operator41/1, Logical Operator42/1
  Logical Operator/1 -> Logical Operator39/1, Logical Operator38/1
  Logical Operator2/1 -> Logical Operator/1
  Logical Operator6/1 -> Logical Operator3/1
  Logical Operator7/1 -> Logical Operator4/1
  Logical Operator8/1 -> Logical Operator5/1
  Decoder_2_to_4/1 -> Logical Operator2/2
  Decoder_2_to_4/2 -> Logical Operator6/2
  Decoder_2_to_4/3 -> Logical Operator7/2
  Decoder_2_to_4/4 -> Logical Operator8/2
  RowAccess(1b)/1 -> Logical Operator2/1, Logical Operator6/1, Logical Operator7/1, Logical Operator8/1

== system Tetris/Display_32x16 ==
  note: Individual words in video memory are interpreted as columns by the Matrix Concatenate block in the following way:
      | - Word with the highest address is interpreted as the left-most column.
      | - Word with the lowest address is interpreted as the right-most column.
      | - MSB bit is interpreted as the top pixel of a particular column.
      | - LSB bit is interpreted as the bottom pixel of a particular column.
      |
      | On screen we want to interpret the words as rows (to correspond to the memory layout) in the following way:
      | - Word with highest address represents top row.
      | - Word with lowest address represents bottom row.
      | - MSB bit represents left-most pixel.
      | - LSB bit represents right-most pixel.
      |
      | To achieve this the Permute Dimensions block is utilized.
  Video(32x16b) : Inport
  Bus Selector1 : BusSelector  OutputSignals=signal1,signal2,signal3,signal4,signal5,signal6,signal7,signal8,signal9,signal10,signal11,signal12,signal13,signal14,signal15,signal16,signal17,signal18,signal19,signal20,signal21,signal22,signal23,signal24,signal25,signal26,signal27,signal28,signal29,signal30,signal31,signal32
  Matrix Concatenate6 : Concatenate  NumInputs=32  Mode=Multidimensional array  ConcatenateDimension=2
  Matrix Viewer2 : dspobslib/Matrix Viewer  ImageParams=off  CMapStr=[0 0.3 0; 0 1 0]  AxisColorbar=on  AxisParams=off  AxisOrigin=Upper left corner  AxisTickMode=Auto  XTickRange=[0 1]  YTickRange=[0 1]  XLabel=X-axis  YLabel=Y-axis  ZLabel=Z-axis  FigPos=[1700 10 200 400]  AxisZoom=on
      settings: YMin=0  YMax=1
  Permute Dimensions : PermuteDimensions
  wires:
  Matrix Concatenate6/1 -> Permute Dimensions/1
  Video(32x16b)/1 -> Bus Selector1/1
  Bus Selector1/9 -> Matrix Concatenate6/9  "<signal9>"
  Bus Selector1/1 -> Matrix Concatenate6/1  "<signal1>"
  Bus Selector1/2 -> Matrix Concatenate6/2  "<signal2>"
  Bus Selector1/32 -> Matrix Concatenate6/32  "<signal32>"
  Bus Selector1/31 -> Matrix Concatenate6/31  "<signal31>"
  Bus Selector1/30 -> Matrix Concatenate6/30  "<signal30>"
  Bus Selector1/29 -> Matrix Concatenate6/29  "<signal29>"
  Bus Selector1/28 -> Matrix Concatenate6/28  "<signal28>"
  Bus Selector1/27 -> Matrix Concatenate6/27  "<signal27>"
  Bus Selector1/26 -> Matrix Concatenate6/26  "<signal26>"
  Bus Selector1/25 -> Matrix Concatenate6/25  "<signal25>"
  Bus Selector1/3 -> Matrix Concatenate6/3  "<signal3>"
  Bus Selector1/4 -> Matrix Concatenate6/4  "<signal4>"
  Bus Selector1/5 -> Matrix Concatenate6/5  "<signal5>"
  Bus Selector1/6 -> Matrix Concatenate6/6  "<signal6>"
  Bus Selector1/7 -> Matrix Concatenate6/7  "<signal7>"
  Bus Selector1/8 -> Matrix Concatenate6/8  "<signal8>"
  Bus Selector1/10 -> Matrix Concatenate6/10  "<signal10>"
  Bus Selector1/11 -> Matrix Concatenate6/11  "<signal11>"
  Bus Selector1/12 -> Matrix Concatenate6/12  "<signal12>"
  Bus Selector1/13 -> Matrix Concatenate6/13  "<signal13>"
  Bus Selector1/14 -> Matrix Concatenate6/14  "<signal14>"
  Bus Selector1/15 -> Matrix Concatenate6/15  "<signal15>"
  Bus Selector1/16 -> Matrix Concatenate6/16  "<signal16>"
  Bus Selector1/17 -> Matrix Concatenate6/17  "<signal17>"
  Bus Selector1/18 -> Matrix Concatenate6/18  "<signal18>"
  Bus Selector1/19 -> Matrix Concatenate6/19  "<signal19>"
  Bus Selector1/20 -> Matrix Concatenate6/20  "<signal20>"
  Bus Selector1/21 -> Matrix Concatenate6/21  "<signal21>"
  Bus Selector1/22 -> Matrix Concatenate6/22  "<signal22>"
  Bus Selector1/23 -> Matrix Concatenate6/23  "<signal23>"
  Bus Selector1/24 -> Matrix Concatenate6/24  "<signal24>"
  Permute Dimensions/1 -> Matrix Viewer2/1

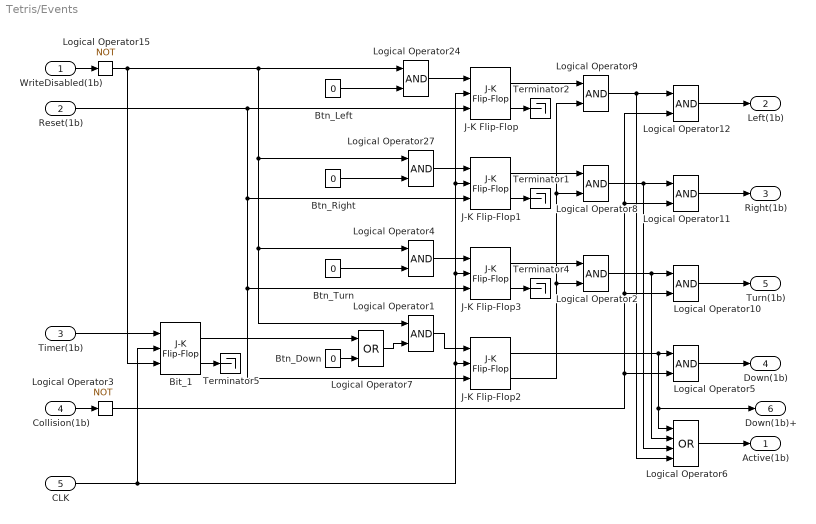
== system Tetris/Events ==
  WriteDisabled(1b) : Inport
  Reset(1b) : Inport  Port=2
  Timer(1b) : Inport  Port=3
  Collision(1b) : Inport  Port=4
  CLK : Inport  Port=5
  Bit_1 : simulink_extras/Flip Flops/J-K Flip-Flop  initial_condition=0
  Btn_Down : Constant  Value=0  OutDataTypeStr=boolean
  Btn_Left : Constant  Value=0  OutDataTypeStr=boolean
  Btn_Right : Constant  Value=0  OutDataTypeStr=boolean
  Btn_Turn : Constant  Value=0  OutDataTypeStr=boolean
  J-K Flip-Flop{,1..3} (4 alike) : simulink_extras/Flip Flops/J-K Flip-Flop  initial_condition=0
  Logical Operator{1..2,4..5,8..12,24,27} (11 alike) : Logic  IconShape=distinctive  AllPortsSameDT=off  OutDataTypeStr=boolean
  Logical Operator15 : Logic  Operator=NOT  Inputs=4  IconShape=distinctive  AllPortsSameDT=off  OutDataTypeStr=boolean
  Logical Operator3 : Logic  Operator=NOT  Inputs=4  IconShape=distinctive  AllPortsSameDT=off  OutDataTypeStr=boolean
  Logical Operator6 : Logic  Operator=OR  Inputs=4  IconShape=distinctive  AllPortsSameDT=off  OutDataTypeStr=boolean
  Logical Operator7 : Logic  Operator=OR  IconShape=distinctive  AllPortsSameDT=off  OutDataTypeStr=boolean
  Terminator{1..2,4..5} (4 alike) : Terminator
  Active(1b) : Outport
  Left(1b) : Outport  Port=2
  Right(1b) : Outport  Port=3
  Down(1b) : Outport  Port=4
  Turn(1b) : Outport  Port=5
  Down(1b)+ : Outport  Port=6
  wires:
  J-K Flip-Flop1/1 -> Logical Operator8/1
  J-K Flip-Flop/2 -> Terminator2/1
  Logical Operator27/1 -> J-K Flip-Flop1/1
  Btn_Right/1 -> Logical Operator27/2
  J-K Flip-Flop1/2 -> Terminator1/1
  CLK/1 -> J-K Flip-Flop3/2, J-K Flip-Flop1/2, J-K Flip-Flop/2, J-K Flip-Flop2/2, Bit_1/2
  Btn_Left/1 -> Logical Operator24/2
  Logical Operator24/1 -> J-K Flip-Flop/1
  J-K Flip-Flop/1 -> Logical Operator9/1
  Btn_Down/1 -> Logical Operator7/2
  J-K Flip-Flop2/1 -> Down(1b)+/1, Logical Operator6/1, Logical Operator5/1
  Logical Operator1/1 -> J-K Flip-Flop2/1
  J-K Flip-Flop3/1 -> Logical Operator2/1
  Logical Operator4/1 -> J-K Flip-Flop3/1
  Reset(1b)/1 -> J-K Flip-Flop/3, J-K Flip-Flop1/3, J-K Flip-Flop2/3, J-K Flip-Flop3/3
  Btn_Turn/1 -> Logical Operator4/2
  WriteDisabled(1b)/1 -> Logical Operator15/1
  J-K Flip-Flop3/2 -> Terminator4/1
  Logical Operator7/1 -> Logical Operator1/2
  Bit_1/1 -> Logical Operator7/1
  Logical Operator8/1 -> Logical Operator11/1, Logical Operator6/3
  Logical Operator9/1 -> Logical Operator6/4, Logical Operator12/1
  Logical Operator2/1 -> Logical Operator6/2, Logical Operator10/1
  Logical Operator15/1 -> Bit_1/3, Logical Operator24/1, Logical Operator27/1, Logical Operator1/1, Logical Operator4/1
  Timer(1b)/1 -> Bit_1/1
  Bit_1/2 -> Terminator5/1
  J-K Flip-Flop2/2 -> Logical Operator9/2, Logical Operator8/2, Logical Operator2/2
  Collision(1b)/1 -> Logical Operator3/1
  Logical Operator5/1 -> Down(1b)/1
  Logical Operator6/1 -> Active(1b)/1
  Logical Operator10/1 -> Turn(1b)/1
  Logical Operator11/1 -> Right(1b)/1
  Logical Operator12/1 -> Left(1b)/1
  Logical Operator3/1 -> Logical Operator5/2, Logical Operator10/2, Logical Operator11/2, Logical Operator12/2
